simulink model "SingleTrack"  (R2021b)
settings: Solver=FixedStepDiscrete  StartTime=0.0  StopTime=tf  RelTol=1e-3
values from neighbouring files (symbols this model uses):
  F0 = zeros(9,1)    [IConditions.m]
  pose0 = [x0, y0, z0, theta0, sigma0, beta0]    [IConditions.m]
  X0 = IConditions()    [SingleTrack_RunSIM.m]
undefined symbols (not defined in the file or in its folder): DiscIntNeverNeededParam
libraries: slpidlib x2, simulink x1
settings Model: Creator=mariotilocca  LastModifiedBy=mariotilocca

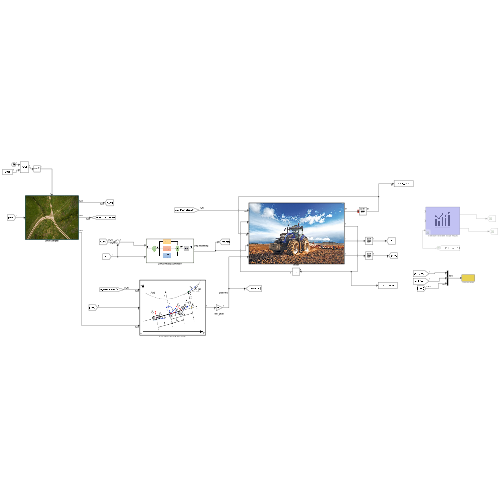
[thumbnail: Simulink's stored preview of the top-level diagram]
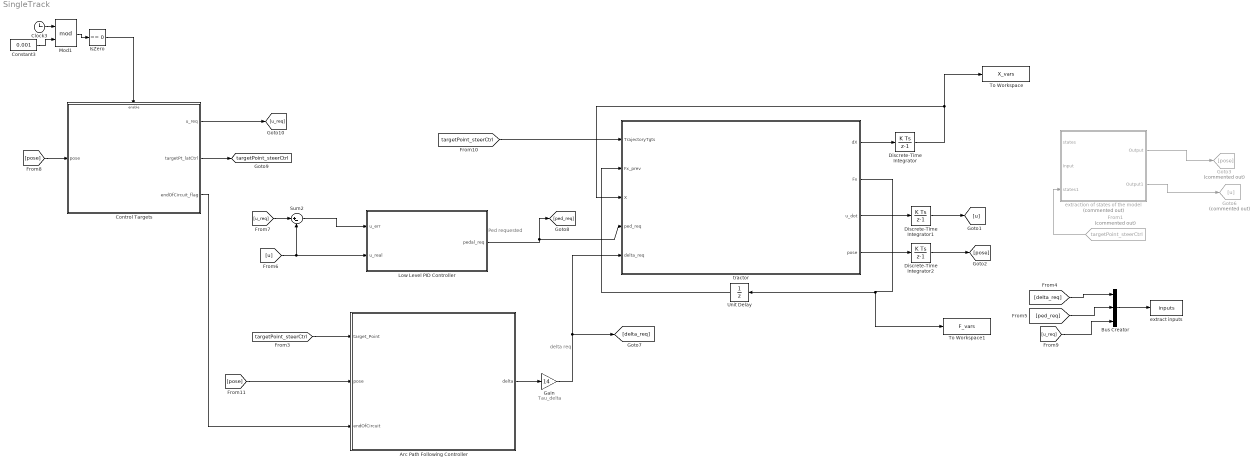
== system SingleTrack ==
  note: Tau_delta
  note: delta req
  note: Ped requested
  Arc Path Following Controller : MATLAB Function  TreatAsAtomicUnit=on
  Bus Creator : BusCreator  Inputs=3
  Clock3 : Clock
  Constant3 : Constant  Value=0.001
  Control Targets : Subsystem
      mask Display: image('$imagefile'); % Use "Edit Image" on toolstrip to change.
  Discrete-Time Integrator : DiscreteIntegrator  gainval=1  InitialCondition=X0  SampleTime=-1  ICPrevOutput=DiscIntNeverNeededParam  ICPrevScaledInput=DiscIntNeverNeededParam
  Discrete-Time Integrator1 : DiscreteIntegrator  gainval=1  InitialCondition=X0(4)  SampleTime=-1  ICPrevOutput=DiscIntNeverNeededParam  ICPrevScaledInput=DiscIntNeverNeededParam
  Discrete-Time Integrator2 : DiscreteIntegrator  gainval=1  InitialCondition=pose0  SampleTime=-1  ICPrevOutput=DiscIntNeverNeededParam  ICPrevScaledInput=DiscIntNeverNeededParam
  From1 : From  Commented=on  GotoTag=targetPoint_steerCtrl  TagVisibility=global
  Gain : Gain  Gain=14
  Goto3 : Goto  Commented=on  GotoTag=pose
  Goto6 : Goto  Commented=on  GotoTag=u
  IsZero : simulink/Logic and Bit Operations/Compare To Zero  relop===  OutDataTypeStr=boolean
  Low Level PID Controller : Subsystem
      mask Display: image('$imagefile'); % Use "Edit Image" on toolstrip to change.
  Mod1 : Math  Operator=mod  SignedPower=on  SaturateOnIntegerOverflow=on
  Sum2 : Sum  Inputs=|+-
  To Workspace : ToWorkspace  VariableName=X_vars  SaveFormat=Timeseries  SampleTime=-1
  To Workspace1 : ToWorkspace  VariableName=F_vars  SaveFormat=Timeseries  SampleTime=-1
  Unit Delay : UnitDelay  InitialCondition=F0  SampleTime=-1  HasFrameUpgradeWarning=on
  extract inputs : ToWorkspace  VariableName=inputs  SaveFormat=Timeseries  SampleTime=-1
  extraction of states of the model : Subsystem  Commented=on
      mask Display: image('$imagefile'); % Use "Edit Image" on toolstrip to change.
  tractor : MATLAB Function  TreatAsAtomicUnit=on
  tag scope: targetPoint_steerCtrl=global
  wires:
  tractor/1(dX) -> Discrete-Time Integrator/1
  Discrete-Time Integrator/1 -> To Workspace/1, tractor/3(X)
  tractor/2(Fx) -> Unit Delay/1, To Workspace1/1
  Bus Creator/1 -> extract inputs/1
  [delta_req] -> Bus Creator/1
  extraction of states of the model/2(Output1) -> Goto6/1
  extraction of states of the model/1(Output) -> Goto3/1
  Low Level PID Controller/1(pedal_req) -> [ped_req], tractor/4(ped_req)
  Gain/1 -> [delta_req], tractor/5(delta_req)
  Sum2/1 -> Low Level PID Controller/1(u_err)
  [u_req] -> Sum2/1
  [u] -> Low Level PID Controller/2(u_real), Sum2/2
  [targetPoint_steerCtrl] -> Arc Path Following Controller/1(target_Point)
  [pose] -> Arc Path Following Controller/2(pose)
  Arc Path Following Controller/1(delta) -> Gain/1
  [ped_req] -> Bus Creator/2
  Clock3/1 -> Mod1/1
  Mod1/1 -> IsZero/1
  Control Targets/2(targetPt_latCtrl) -> [targetPoint_steerCtrl]
  [pose] -> Control Targets/1(pose)
  Constant3/1 -> Mod1/2
  Control Targets/1(u_req) -> [u_req]
  Control Targets/3(endOfCircuit_flag) -> Arc Path Following Controller/3(endOfCircuit)
  IsZero/1 -> Control Targets/Enable
  [u_req] -> Bus Creator/3
  [targetPoint_steerCtrl] -> tractor/1(TrajectoryTgts)
  From1/1 -> extraction of states of the model/3(states1)
  tractor/3(u_dot) -> Discrete-Time Integrator1/1
  Discrete-Time Integrator1/1 -> [u]
  tractor/4(pose) -> Discrete-Time Integrator2/1
  Discrete-Time Integrator2/1 -> [pose]
  Unit Delay/1 -> tractor/2(Fx_prev)

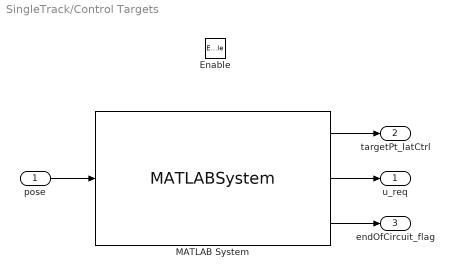
== system SingleTrack/Control Targets ==
  pose : Inport
  Enable : EnablePort
  MATLAB System : MATLABSystem  System=setControlTargets  purePursuit_lookAhead=5  SimulateUsing=Code generation
      mask Type: setControlTargets
      mask Display:
      | disp('setControlTargets');
      | port_label('input',1,'vehPose');
      | port_label('output',1,'targetPoint_latControl');
      | port_label('output',2,'speed_req');
      | port_label('output',3,'endOfCircuit');
  u_req : Outport  VectorParamsAs1DForOutWhenUnconnected=off
  targetPt_latCtrl : Outport  Port=2  VectorParamsAs1DForOutWhenUnconnected=off
  endOfCircuit_flag : Outport  Port=3  VectorParamsAs1DForOutWhenUnconnected=off
  wires:
  pose/1 -> MATLAB System/1
  MATLAB System/2 -> u_req/1
  MATLAB System/1 -> targetPt_latCtrl/1
  MATLAB System/3 -> endOfCircuit_flag/1

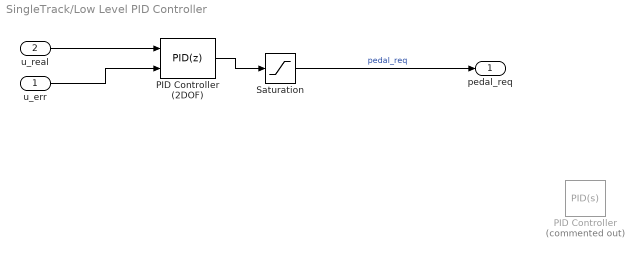
== system SingleTrack/Low Level PID Controller ==
  u_err : Inport
  u_real : Inport  Port=2
  PID Controller : slpidlib/PID Controller  Commented=on  Controller=PID  Form=Parallel  TimeDomain=Continuous-time  UseExternalTs=off  SampleTime=-1  IntegratorMethod=Forward Euler  FilterMethod=Forward Euler  ControllerParametersSource=internal  P=1  I=1  D=0  UseFilter=on  N=100  TunerSelectOption=Transfer Function Based (PID Tuner App)  InitialConditionSource=internal  InitialConditionForIntegrator=0  InitialConditionForFilter=0  DifferentiatorICPrevScaledInput=0  ExternalReset=none  TrackingMode=off  Kt=1  LimitOutput=off  SatLimitsSource=internal  UpperSaturationLimit=inf  LowerSaturationLimit=-inf  LinearizeAsGain=on  AntiWindupMode=none  Kb=1  POutMin=[]  POutMax=[]  IOutMin=[]  IOutMax=[]  DOutMin=[]  DOutMax=[]  NOutMin=[]  NOutMax=[]  SumOutMin=[]  SumOutMax=[]  SaturationOutMin=[]  SaturationOutMax=[]  PParamMin=[]  PParamMax=[]  IParamMin=[]  IParamMax=[]  DParamMin=[]  DParamMax=[]  NParamMin=[]  NParamMax=[]  KbParamMin=[]  KbParamMax=[]  KtParamMin=[]  KtParamMax=[]  KbOutMin=[]  KbOutMax=[]  KtOutMin=[]  KtOutMax=[]  IntegratorOutMin=[]  IntegratorOutMax=[]  FilterOutMin=[]  FilterOutMax=[]  SumI1OutMin=[]  SumI1OutMax=[]  SumI2OutMin=[]  SumI2OutMax=[]  SumI3OutMin=[]  SumI3OutMax=[]  SumI4OutMin=[]  SumI4OutMax=[]  SumDOutMin=[]  SumDOutMax=[]  DifferentiatorOutMin=[]  DifferentiatorOutMax=[]  FilterDiffOutCoefMin=[]  FilterDiffOutCoefMax=[]  ReciprocalOutMin=[]  ReciprocalOutMax=[]  SumDenOutMin=[]  SumDenOutMax=[]  SumNumOutMin=[]  SumNumOutMax=[]  DivideOutMin=[]  DivideOutMax=[]  UdiffTsProdOutMin=[]  UdiffTsProdOutMax=[]  NTsProdOutMin=[]  NTsProdOutMax=[]  UintegralTsProdOutMin=[]  UintegralTsProdOutMax=[]  UngainTsProdOutMin=[]  UngainTsProdOutMax=[]  IntegratorContinuousStateAttributes=''  IntegratorStateMustResolveToSignalObject=off  IntegratorRTWStateStorageClass=Auto  FilterContinuousStateAttributes=''  FilterStateMustResolveToSignalObject=off  FilterRTWStateStorageClass=Auto  ParallelPVariant=InternalParameters  IdealPVariant=Disabled  IVariant=InternalParameters  DVariant=InternalParameters  IntegratorVariant=Continuous  SatVariant=Disabled  AWVariant=Passthrough  PCopyVariant=Disabled  TRVariant=Disabled  FdbkBlocksVariant=Forward  IdealPFdbkVariant=Disabled  SatFdbkVariant=Disabled  DerivativeFilterVariant=ContFilter  NVariant=InternalParameters  NCopyVariant=Disabled  FilterICVariant=InternalICsFilter  IntegratorICVariant=InternalICs  ExternalResetVariant=Disabled  TRSumVariant=Passthrough  SumFdbkVariant=Disabled  SumVariant=Sum_PID  TsampFilterVariant=InternalTs  TsampNgainVariant=Passthrough  TsampIntegralVariant=Passthrough  ExternalSaturationOutDataTypeStr=Inherit: Same as second input
  PID Controller (2DOF) : slpidlib/PID Controller (2DOF)  Controller=PID  Form=Parallel  TimeDomain=Discrete-time  UseExternalTs=off  SampleTime=-1  IntegratorMethod=Forward Euler  FilterMethod=Forward Euler  ControllerParametersSource=internal  P=22  I=2.5  D=3  UseFilter=on  N=100  b=1  c=1  TunerSelectOption=Transfer Function Based (PID Tuner App)  InitialConditionSource=internal  InitialConditionForIntegrator=0  InitialConditionForFilter=0  DifferentiatorICPrevScaledInput=0  ExternalReset=none  TrackingMode=off  Kt=1  LimitOutput=off  SatLimitsSource=internal  UpperSaturationLimit=inf  LowerSaturationLimit=-inf  LinearizeAsGain=on  AntiWindupMode=none  Kb=1  POutMin=[]  POutMax=[]  IOutMin=[]  IOutMax=[]  DOutMin=[]  DOutMax=[]  NOutMin=[]  NOutMax=[]  bOutMin=[]  bOutMax=[]  cOutMin=[]  cOutMax=[]  SumOutMin=[]  SumOutMax=[]  SaturationOutMin=[]  SaturationOutMax=[]  PParamMin=[]  PParamMax=[]  IParamMin=[]  IParamMax=[]  DParamMin=[]  DParamMax=[]  NParamMin=[]  NParamMax=[]  bParamMin=[]  bParamMax=[]  cParamMin=[]  cParamMax=[]  KbParamMin=[]  KbParamMax=[]  KtParamMin=[]  KtParamMax=[]  KbOutMin=[]  KbOutMax=[]  KtOutMin=[]  KtOutMax=[]  IntegratorOutMin=[]  IntegratorOutMax=[]  FilterOutMin=[]  FilterOutMax=[]  SumI1OutMin=[]  SumI1OutMax=[]  SumI2OutMin=[]  SumI2OutMax=[]  SumI3OutMin=[]  SumI3OutMax=[]  SumI4OutMin=[]  SumI4OutMax=[]  SumDOutMin=[]  SumDOutMax=[]  Sum1OutMin=[]  Sum1OutMax=[]  Sum2OutMin=[]  Sum2OutMax=[]  Sum3OutMin=[]  Sum3OutMax=[]  DifferentiatorOutMin=[]  DifferentiatorOutMax=[]  FilterDiffOutCoefMin=[]  FilterDiffOutCoefMax=[]  ReciprocalOutMin=[]  ReciprocalOutMax=[]  SumDenOutMin=[]  SumDenOutMax=[]  SumNumOutMin=[]  SumNumOutMax=[]  DivideOutMin=[]  DivideOutMax=[]  UdiffTsProdOutMin=[]  UdiffTsProdOutMax=[]  NTsProdOutMin=[]  NTsProdOutMax=[]  UintegralTsProdOutMin=[]  UintegralTsProdOutMax=[]  UngainTsProdOutMin=[]  UngainTsProdOutMax=[]  IntegratorContinuousStateAttributes=''  IntegratorStateMustResolveToSignalObject=off  IntegratorRTWStateStorageClass=Auto  FilterContinuousStateAttributes=''  FilterStateMustResolveToSignalObject=off  FilterRTWStateStorageClass=Auto  ParallelPVariant=InternalParameters  IdealPVariant=Disabled  IVariant=InternalParameters  DVariant=InternalParameters  bVariant=InternalParameters  cVariant=InternalParameters  IntegratorVariant=Discrete  SatVariant=Disabled  AWVariant=Passthrough  PCopyVariant=Disabled  TRVariant=Disabled  FdbkBlocksVariant=Forward  IdealPFdbkVariant=Disabled  SatFdbkVariant=Disabled  DerivativeFilterVariant=ForwardEulerFilter  NVariant=InternalParameters  NCopyVariant=Disabled  FilterICVariant=InternalICsFilter  IntegratorICVariant=InternalICs  ExternalResetVariant=Disabled  TRSumVariant=Passthrough  SumFdbkVariant=Disabled  SumVariant=Sum_PID  TsampFilterVariant=InternalTs  TsampNgainVariant=Passthrough  TsampIntegralVariant=Passthrough  ExternalSaturationOutDataTypeStr=Inherit: Same as second input
      settings: SourceProductBaseCode=SL
  Saturation : Saturate  UpperLimit=1  LowerLimit=-1
  pedal_req : Outport  VectorParamsAs1DForOutWhenUnconnected=off
  wires:
  Saturation/1 -> pedal_req/1  "pedal_req"
  u_real/1 -> PID Controller (2DOF)/1
  u_err/1 -> PID Controller (2DOF)/2
  PID Controller (2DOF)/1 -> Saturation/1

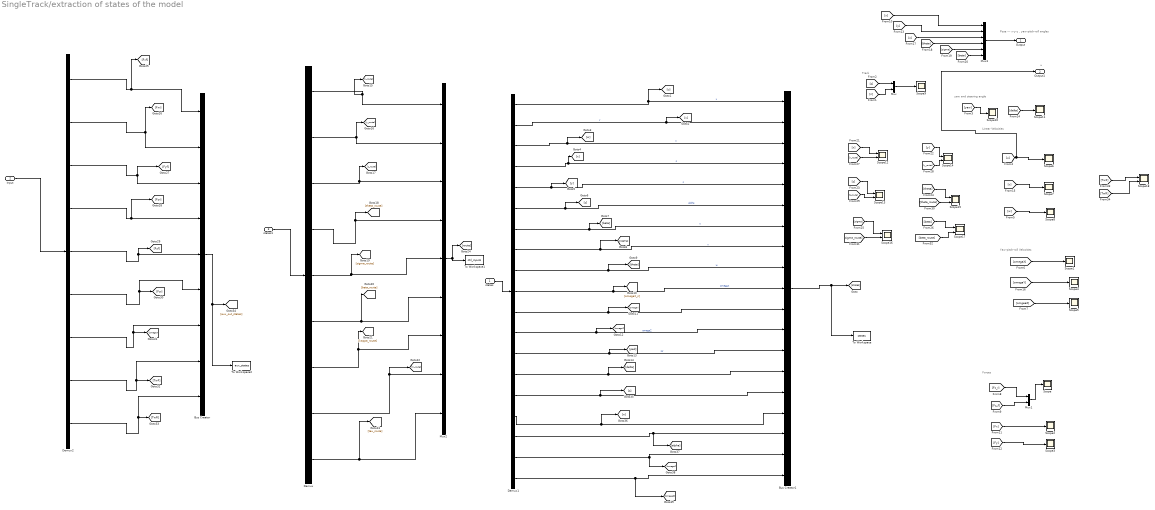
== system SingleTrack/extraction of states of the model ==
  note: u
  note: Pose --- x-y-z , yaw-pitch-roll angles
  note: yaw and steering angle
  note: Track
  note: Forces
  note: Yaw-pitch-roll Velocities
  note: Linear Velocities
  states : Inport
  Input : Inport  Port=2
  states1 : Inport  Port=3
  Bus Creator : BusCreator  Inputs=9
  Bus Creator1 : BusCreator  Inputs=19
  Demux : Demux  Outputs=9
  Demux1 : Demux  Outputs=19
  Demux2 : Demux  Outputs=9  BusSelectionMode=on
  Mux : Mux  Inputs=2
  Mux1 : Mux  Inputs=2
  Mux2 : Mux  Inputs=9
  Mux3 : Mux  Inputs=6
  Scope{,1..11} (12 alike) : Scope
  Scope{12..18} (7 alike) : Scope  NumInputPorts=2
  To Workspace : ToWorkspace  VariableName=states  SaveFormat=Timeseries  SampleTime=-1
  To Workspace1 : ToWorkspace  VariableName=ctrl_inputs  SaveFormat=Timeseries  SampleTime=-1
  To Workspace2 : ToWorkspace  VariableName=aux_states  SaveFormat=Timeseries  SampleTime=-1
  Output : Outport
  Output1 : Outport  Port=2
  wires:
  states/1 -> Demux1/1
  [s] -> Mux/1
  [n] -> Mux/2
  [Fz_r] -> Mux1/1
  [Fz_f] -> Mux1/2
  Mux1/1 -> Scope/1
  [Fx] -> Scope2/1
  [Fy] -> Scope3/1
  [omegaX] -> Scope1/1
  [omegaY] -> Scope4/1
  [omgeaZ] -> Scope5/1
  [u] -> Scope6/1, Output1/1
  [v] -> Scope7/1
  [w] -> Scope8/1
  Mux/1 -> Scope9/1
  [yaw] -> Scope10/1
  [delta] -> Scope11/1
  Mux3/1 -> Output/1
  states1/1 -> Demux/1
  Demux/1 -> [x_route], Mux2/1
  Demux/2 -> [y_route], Mux2/2
  Demux/3 -> [z_route], Mux2/3
  Demux/4 -> [theta_route], Mux2/4
  Demux/5 -> [sigma_route], Mux2/5
  Demux/6 -> [beta_route], Mux2/6
  Demux/7 -> [kappa_route], Mux2/7
  Demux/8 -> [ni_route], Mux2/8
  Demux/9 -> Mux2/9, [tau_route]
  Mux2/1 -> [route], To Workspace1/1
  Demux2/1 -> [Fxf], Bus Creator/1
  Demux2/2 -> [Fxr], Bus Creator/2
  Demux2/3 -> [Fyf], Bus Creator/3
  Demux2/4 -> [Fyr], Bus Creator/4
  Demux2/5 -> [Fzf], Bus Creator/5
  Demux2/6 -> Bus Creator/6, [Fzr]
  Demux2/7 -> Bus Creator/7, [omegaX]
  Demux2/8 -> Bus Creator/8, [TwF]
  Demux2/9 -> Bus Creator/9, [TwR]
  Input/1 -> Demux2/1
  Bus Creator/1 -> To Workspace2/1, [aux_out_states]
  Demux1/1 -> [u], Bus Creator1/1  "x"
  Demux1/2 -> [v], Bus Creator1/2  "y"
  Demux1/3 -> [w], Bus Creator1/3  "z"
  Demux1/4 -> [x], Bus Creator1/4  "s"
  Demux1/5 -> [y], Bus Creator1/5  "n"
  Demux1/6 -> [z], Bus Creator1/6  "alpha"
  Demux1/7 -> [beta], Bus Creator1/7  "u"
  Demux1/8 -> [sigma], Bus Creator1/8  "v"
  Demux1/9 -> [theta], Bus Creator1/9  "w"
  Demux1/10 -> [omegaX_n], Bus Creator1/10  "omegaX"
  Demux1/11 -> [omegaY], Bus Creator1/11
  Demux1/12 -> [omegaZ], Bus Creator1/12  "omegaZ"
  Demux1/13 -> [ped], Bus Creator1/13  "Nr"
  Demux1/14 -> [delta], Bus Creator1/14
  Demux1/15 -> [s], Bus Creator1/15
  Demux1/16 -> [n], Bus Creator1/16
  Demux1/17 -> [alpha], Bus Creator1/17
  Demux1/18 -> Bus Creator1/18, [omegaF]
  Demux1/19 -> [omegaR], Bus Creator1/19
  Bus Creator1/1 -> To Workspace/1, [states]
  [x] -> Mux3/1
  [y] -> Mux3/2
  [z] -> Mux3/3
  [theta] -> Mux3/4
  [sigma] -> Mux3/5
  [beta] -> Mux3/6
  [x] -> Scope12/1
  [x_route] -> Scope12/2
  [z] -> Scope13/1
  [z_route] -> Scope13/2
  [y] -> Scope14/1
  [y_route] -> Scope14/2
  [theta] -> Scope15/1
  [theta_route] -> Scope15/2
  [sigma] -> Scope16/1
  [sigma_route] -> Scope16/2
  [beta] -> Scope17/1
  [beta_route] -> Scope17/2
  [TwF] -> Scope18/1
  [TwR] -> Scope18/2

== matlab function SingleTrack/tractor ==
  data: TrajectoryTgts input; Fx_prev input; X input; ped_req input; dX output; delta_req input; Fx output; u_dot output; pose output
function [dX, Fx, u_dot, pose] = tractor(TrajectoryTgts, Fx_prev, X, ped_req, delta_req)
%% -- INPUTS OF THE MODEL --
%   kappa --> road heading at road poit 
%   ni --> road slope at road point 
%   tau --> road banking at road point 
%   dxPRev --> previous vehicle dynamics state derivatives 
%   X --> vehicle dynamics state at previous time step 
%  ped_req --> requested longitudinal velocity 
%   omega_delta --> steering speed 
%
%
%% Vehicle Data 


M = 1014; % mass of the vhicle 

a = 1.2; % rear axle length from centre of mass 
b = 1.29; % front axle length from centre of mass 
h = 0.5; % height from the terrain w.r.t. centre of mass 

Kr = 90232.5227453858; % side slip cornering stiffness - rear
Kf = 67740.0047457928; % side slip cornering stiffness - front 

Skf = 82216.6666666667;
Skr = 41727.2727272727; % rear longitudinal slip coefficient 

Iyy =50; % pitch inertia [kg*m^2]
Ixz =1950; % cross inertia 
Izz =1730; % yaw inertia 
Ixx = 590; % roll inertia 

dt = 0.001; % time step 
g = 9.81; 

tau_D =14;
tau_H = 0.03;

tau_ped= 0.03; 

%% Trajectory params extraction 

kappa = TrajectoryTgts(7);
ni =  TrajectoryTgts(8);
tau = TrajectoryTgts(9);

sigma =  TrajectoryTgts(5);
beta =  TrajectoryTgts(6);



%% Variables definition 

% ---- init conditions structure ----- % 

%  cond = [x0, y0, z0, u0, v0, w0, beta0, sigma0, theta0, omegaX0, omegaY0, omegaZ0, pedal0, delta0, s0, n0, alpha0, omegaFront0, omegaRear0]; 



% dX(1) = u_dot ;
% dX(2) = v_dot;
% dX(3) = w_dot;

u = X(4);

disp("------- tractor main framework --------")
disp("longitudinal velocity")
disp(u)
disp(" ********************************")


v = X(5);
w = X(6);

% dX(4) = u;
% dX(5) = v;
% dX(6) = w;

x = X(1);
y = X(2);
z = X(3);

omegaX = X(10);
omegaY = X(11);
omegaZ = X(12);

ped = X(13);
delta = X(14);
s = X(15);
n = X(16);

alpha = X(17);
omegaFront = X(18);
omegaRear = X(19);


% dX(7) = omegaX;
% dX(8) = omegaY;
% dX(9) = omegaZ;

% dX(10) = omegaXdot;
% dX(11) = omegaYdot;
% dX(12) = omegaZdot;
% dX(13) = ped_dot;
% dX(14) = delta_dot;
% dX(15) = s_dot;
% dX(16) = n_dot;
% dX(17) = alpha_dot; 
% dX(18) = omegaFront_dot;
% dX(19) = omegaRear_dot; 
% 




Fxf = Fx_prev(1); % init forces ? 
Fxr = Fx_prev(2);
omegaXprev = Fx_prev(7);


% s = X(1) ;  % road position
% n = X(2) ; % road lateral coordinates 
% alpha = X(3); % yaw angle 
% u = X(4);  % longit velocity 
% v = X(5); % lateral velocity 
% w = X(6); % vertical veloctiy 
% omegaX = X(7); % roll rot velocity 
% omegaY = X(8); % pitch rot velocity [rad/s]
% omegaZ = X(9) ; % yaw rot velocity 
% Nr = X(10) ; % rear tire load 
% Nf = X(11); % front tire load 
% S = X(12); % longitudinal forces Fxf + Fxr 
% delta = X(13) ; % steering angle front wheel 


%% output initialization

dX = zeros(19,1);
Fx = zeros(9,1);
pose = zeros(6,1); 



 %%  Trorques model
    
    maxTorque = 476; 
    brakeRatio = 0.5 ; 
    brakeTorqueMax = maxTorque * 2; 
    
    % Driving torques at the wheels & Acceleration 
    Tm_req = posPart(ped)*maxTorque;  %

    % tractive torques 
    TwFtraction = MotorModel(Tm_req,true);
    TwRtraction = MotorModel(Tm_req,false);
     
    
    % braking torques 

    TbR_req = -negPart(ped)*brakeTorqueMax*(1-brakeRatio);
    TbF_req = -negPart(ped)*brakeTorqueMax*brakeRatio;
    
    % Front wheels braking model  - same for both front and rear 
    [TwFbrake,TwRbrake] = BrakeModel(TbF_req,TbR_req,omegaFront,omegaRear);
    
    
    % The total torque for each wheel is the algebraic sum of motor and brake torques
    TwF = TwFtraction + TwFbrake;
    TwR = TwRtraction + TwRbrake;
    

%% Auxiliary models 

omegaFront_dot = wheelRotA(Fxf, true, TwF); % wheel accelerations 
omegaRear_dot = wheelRotA(Fxr, false, TwR);



[Fx_new, Fy_new, Fz_new] = Brush_tyre_model(u, v, delta, omegaZ, omegaFront, omegaRear);  %  add wheel torques to wheel eqs. 

disp("new force longit")
disp(Fx_new)

Fxf = Fx_new(1);
Fxr = Fx_new(2);

Fyf = Fy_new(1);
Fyr = Fy_new(2);

Fzf = Fz_new(1);
Fzr = Fz_new(2);


%% Model equations 


%equations:

%20a
s_dot = (u*cos(alpha)-v*sin(alpha)/(1-n*kappa));


%20b
n_dot = u*sin(alpha)+v*cos(alpha);

%20c
alpha_dot = omegaZ - kappa *(u*cos(alpha)-v*sin(alpha)/(1-n*kappa)); % relative yaw velocity 
%% positioning
% 8a 
u = (1-n*kappa)*s_dot *cos(alpha) + n_dot*sin(alpha); % x- axis position  -- velocity ? 

% 8b
v = -(1-n*kappa)*s_dot *sin(alpha) + n_dot*cos(alpha); % y-

% 8c 
w = n*tau*s_dot; % z axis position 

%% yaw -pitch - roll angles 

%9a
omegaX = (tau*cos(alpha)+ni*sin(alpha))*s_dot; % roll velocity

%9b
omegaY = (-tau*sin(alpha)+ni*cos(alpha))*s_dot; % pitch velocity 


%9c 
omegaZ = kappa*s_dot + alpha_dot;  % yaw velocity 

%% accelerations 


% yaw -pitch - (roll ) 

omegaYdot = (Ixz*omegaZ^2 - omegaX*(Ixx - Izz)*omegaZ + Fzf*a - Fzr*b + h*(Fxf + Fxr - Fyf*delta))/Iyy;


omegaZdot = ((-b*Fyr + a*(Fyf - Fxf*delta))) / Izz; 

omegaXdot = (omegaX - omegaXprev) / dt ; 



 % x-y-z
 u_dot = (Fxf + Fxr - Fyf*delta + M*(beta*sin(alpha) - sigma*cos(alpha)) + M*(omegaZ*v - omegaY*w) + M*h*(omegaYdot + omegaX*omegaZ))/M; 

 v_dot = (Fyf + Fyr - Fxf*delta - M*(omegaZ*u - omegaX*w) - M*h*(omegaXdot - omegaY*omegaZ) + M*g*(beta*cos(alpha) + sigma*sin(alpha)))/M; 

 w_dot = -(Fzf + Fzr - M*g - M*(omegaY*u - omegaX*v))/M; 


%%

% 15 

 % Longitudinal force deriv  --- mass * longitudinal jerk -- probably not needed 
delta_dot    = (-delta * tau_D + delta_req) / tau_D / tau_H; % steering speed (rad/s) 

ped_dot = (ped_req - ped) / tau_ped;

%% -- Output format 


% ---- output to be integrated --- %

dX(1) = u_dot ;
dX(2) = v_dot;
dX(3) = w_dot;
dX(4) = u;
dX(5) = v;
dX(6) = w;
dX(7) = omegaX;
dX(8) = omegaY;
dX(9) = omegaZ;
dX(10) = omegaXdot;
dX(11) = omegaYdot;
dX(12) = omegaZdot;
dX(13) = ped_dot;
dX(14) = delta_dot;
dX(15) = s_dot;
dX(16) = n_dot;
dX(17) = alpha_dot; 
dX(18) = omegaFront_dot;
dX(19) = omegaRear_dot; 


% ----- output not to be integrated ----- %


Fx(1) = Fxf;
Fx(2) = Fxr;
Fx(3) = Fyf;
Fx(4) = Fyr;
Fx(5) = Fzf;
Fx(6) = Fzr;
Fx(7) = omegaX;
Fx(8) = TwF; 
Fx(9) = TwR; 


 %                                                                                                                      

pose(1) = u; % x
pose(2) = v; % y
pose(3) = w;  % z
pose(4) = omegaZ; % theta 
pose(5) = omegaY;  % sigma
pose(6) = omegaX; % beta


end

== matlab function SingleTrack/Arc Path Following Controller ==
  data: target_Point input; delta output; pose input; endOfCircuit input
function delta = arcPathFollowController(target_Point, pose, endOfCircuit)
  
    % Load vehicle params
    a = 1.2;
    b = 1.29;
    L  = a + b;  % [m] vehicle wheelbase
    
    % Current vehicle center of mass pose 
    x_C     = pose(1);
    y_C     = pose(2);
    theta_C = pose(4);  % vehicle attitude (in radians)
    
    %rmat = [cos(theta_C) -sin(theta_C)  0; sin(theta_C) cos(theta_C) 0; 0 0 1];
   %rmat = [cos(theta_C) sin(theta_C); -sin(theta_C) cos(theta_C)];
   %BackP = [x_C y_C] +rmat *[-Lr 0] ; %eul2rotm([0,0,theta_C], "XYZ") * [-Lr;0;0];
    
  %P = [target_Point(1) ; target_Point(2) ] + rmat *   BackP;
if (~endOfCircuit)
   rmat = [cos(theta_C) -sin(theta_C); sin(theta_C) cos(theta_C)] ;
   
   P = ([target_Point(1)  target_Point(2)  ] -[x_C  y_C ]) *rmat; 
    xd = P(1)+b; 
    yd = P(2);
    lam = atan(yd/xd);
    R = sqrt(xd^2+yd^2)/(2*sin(lam));

    delta = atan(L/R);
else 
    delta =0;
end 
    

end
